simulink model "ex1_4"  (Simulink 8.1)
settings: Solver=ode45  StartTime=0.0  StopTime=40  RelTol=1e-3
libraries: simulink x4
settings Model: Creator=Daniel Leal Sousa  LastModifiedBy=Nelson
settings DataIOCC: SignalLoggingSaveFormat=Dataset
settings OptimizationCC: ExpressionDepthLimit=128
settings DebuggingCC: UnderspecifiedInitializationDetection=Simplified  MergeDetectMultiDrivingBlocksExec=error  SolverPrmCheckMsg=none  FcnCallInpInsideContextMsg=EnableAllAsError  FrameProcessingCompatibilityMsg=error  StateNameClashWarn=none
settings GRTTargetCC: CodeReplacementLibrary=None  CombineOutputUpdateFcns=on  CPPClassGenCompliant=on  GRTInterface=off

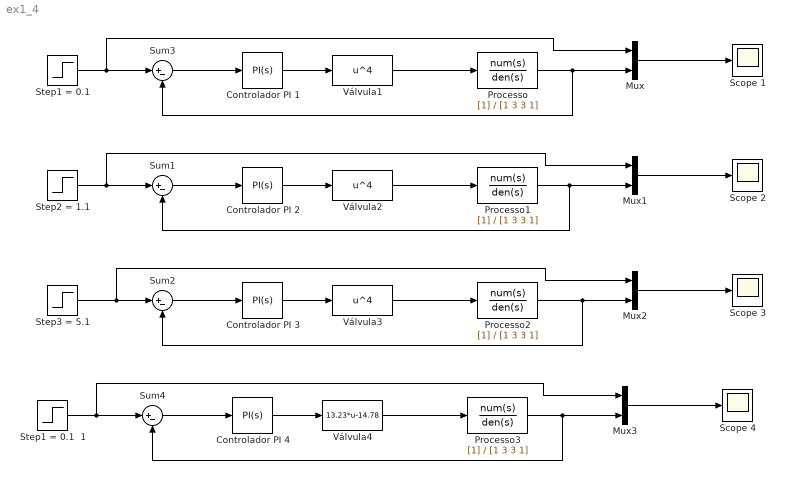
== system ex1_4 ==
  Controlador PI {1..4} (4 alike) : simulink/Continuous/PID Controller  Controller=PI  TimeDomain=Continuous-time  SampleTime=-1  IntegratorMethod=Forward Euler  FilterMethod=Forward Euler  Form=Parallel  P=0.15  I=0.15  D=0  N=100  InitialConditionSource=internal  InitialConditionForIntegrator=0  InitialConditionForFilter=0  ExternalReset=none  LimitOutput=off  UpperSaturationLimit=inf  LowerSaturationLimit=-inf  LinearizeAsGain=on  AntiWindupMode=none  Kb=1  TrackingMode=off  Kt=1  PParamMin=[]  PParamMax=[]  IParamMin=[]  IParamMax=[]  DParamMin=[]  DParamMax=[]  NParamMin=[]  NParamMax=[]  KbParamMin=[]  KbParamMax=[]  KtParamMin=[]  KtParamMax=[]  POutMin=[]  POutMax=[]  IOutMin=[]  IOutMax=[]  DOutMin=[]  DOutMax=[]  NOutMin=[]  NOutMax=[]  KbOutMin=[]  KbOutMax=[]  KtOutMin=[]  KtOutMax=[]  IntegratorOutMin=[]  IntegratorOutMax=[]  FilterOutMin=[]  FilterOutMax=[]  SumOutMin=[]  SumOutMax=[]  SumI1OutMin=[]  SumI1OutMax=[]  SumI2OutMin=[]  SumI2OutMax=[]  SumI3OutMin=[]  SumI3OutMax=[]  SumDOutMin=[]  SumDOutMax=[]  SaturationOutMin=[]  SaturationOutMax=[]  IntegratorContinuousStateAttributes=''  IntegratorStateMustResolveToSignalObject=off  IntegratorRTWStateStorageClass=Auto  FilterContinuousStateAttributes=''  FilterStateMustResolveToSignalObject=off  FilterRTWStateStorageClass=Auto
  Mux{,1..3} (4 alike) : Mux  Inputs=2
  Processo{,1..3} (4 alike) : TransferFcn  Denominator=[1 3 3 1]
  Scope {1..4} (4 alike) : Scope
      Scope 1 settings: SaveName=saida1
      Scope 2 settings: SaveName=saida2
      Scope 3 settings: SaveName=saida3
      Scope 4 settings: SaveName=output
  "Step1 = 0.1  " : Step  Time=0  After=0.3  SampleTime=0
  Step1 = 0.1  1 : Step  Time=0  After=0.3  SampleTime=0
  Step2 = 1.1 : Step  Time=0  After=1.1  SampleTime=0
  Step3 = 5.1 : Step  Time=0  After=5.1  SampleTime=0
  Sum{1..4} (4 alike) : Sum  Inputs=|+-
  Válvula1 : Fcn  Expr=u^4
  Válvula2 : Fcn  Expr=u^4
  Válvula3 : Fcn  Expr=u^4
  Válvula4 : Fcn  Expr=13.23*u-14.78
  wires:
  "Step1 = 0.1  "/1 -> Mux/1, Sum3/1
  Step2 = 1.1/1 -> Mux1/1, Sum1/1
  Step3 = 5.1/1 -> Mux2/1, Sum2/1
  Sum3/1 -> Controlador PI 1/1
  Sum1/1 -> Controlador PI 2/1
  Sum2/1 -> Controlador PI 3/1
  Controlador PI 1/1 -> Válvula1/1
  Controlador PI 2/1 -> Válvula2/1
  Controlador PI 3/1 -> Válvula3/1
  Válvula1/1 -> Processo/1
  Válvula2/1 -> Processo1/1
  Válvula3/1 -> Processo2/1
  Processo/1 -> Mux/2, Sum3/2
  Processo1/1 -> Mux1/2, Sum1/2
  Processo2/1 -> Mux2/2, Sum2/2
  Mux/1 -> Scope 1/1
  Mux1/1 -> Scope 2/1
  Mux2/1 -> Scope 3/1
  Step1 = 0.1  1/1 -> Mux3/1, Sum4/1
  Sum4/1 -> Controlador PI 4/1
  Controlador PI 4/1 -> Válvula4/1
  Válvula4/1 -> Processo3/1
  Processo3/1 -> Mux3/2, Sum4/2
  Mux3/1 -> Scope 4/1
